simulink model "SMC_implementacion"  (R2024a)
settings: Solver=FixedStepAuto  StartTime=0.0  StopTime=inf  RelTol=1e-3  EnableMultiTasking=on
undefined symbols (not defined in the file): a, A_d, B_d, beta, C_d, L_d, theta_ref
libraries: arduinolib x2, eeLuenbergerObserver x1
settings Model: ExtModeTrigDuration=2  Creator=chris  LastModifiedBy=alfar
settings OptimizationCC: EnhancedBackFolding=on  PassReuseOutputArgsThreshold=0  MaxStackSize=64  OptimizeBlockOrder=speed  DifferentSizesBufferReuse=on  OptimizationCustomize=off
settings DebuggingCC: ParameterTunabilityLossMsg=error
settings HardwareCC: ProdBitPerInt=16  ProdBitPerPointer=16  ProdBitPerSizeT=16  ProdBitPerPtrDiffT=16  ProdLargestAtomicFloat=None  ProdWordSize=8  ProdHWDeviceType=Atmel->AVR  UseEmbeddedCoderFeatures=off  UseSimulinkCoderFeatures=off
settings SFSimCC: MATLABDynamicMemAlloc=off
settings RTWCC: Description=Embedded Coder  SystemTargetFile=ert.tlc  HardwareBoard=Arduino Mega 2560  TemplateMakefile=ert_default_tmf  RTWVerbose=off  Toolchain=Arduino AVR  BuildConfiguration=Faster Runs  GPUComputeCapability=3.5
settings CodeAppCC: ForceParamTrailComments=on  OperatorAnnotations=on  MangleLength=10
settings ERTTargetCC: ERTCustomFileBanners=off  SupportContinuousTime=on  SupportNonInlinedSFcns=on  RemoveResetFunc=off  SupportVariableSizeSignals=on  ModelStepFunctionPrototypeControlCompliant=off  ExtMode=on  ExtModeTransport=3  ExtModeStaticAlloc=on  ExtModeAutomaticAllocSize=off  ExtModeStaticAllocSize=2048  ExtModeMexFile=ext_xcp  ExtModeMexArgs=0 6 921600  ExtModeIntrfLevel=Level2 - Open  ERTSrcFileBannerTemplate=codertarget_code_template.cgt  ERTHdrFileBannerTemplate=codertarget_code_template.cgt  ERTDataSrcFileTemplate=codertarget_code_template.cgt  ERTDataHdrFileTemplate=codertarget_code_template.cgt

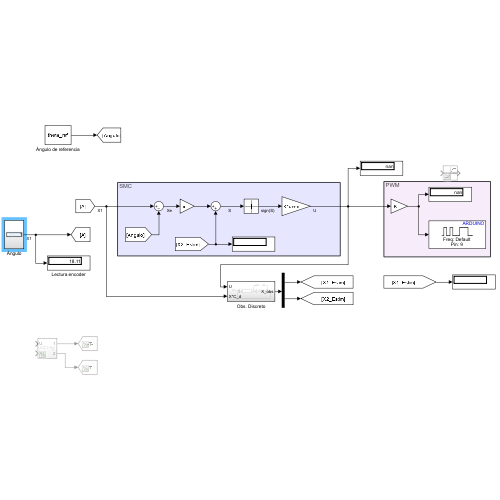
[thumbnail: Simulink's stored preview of the top-level diagram]
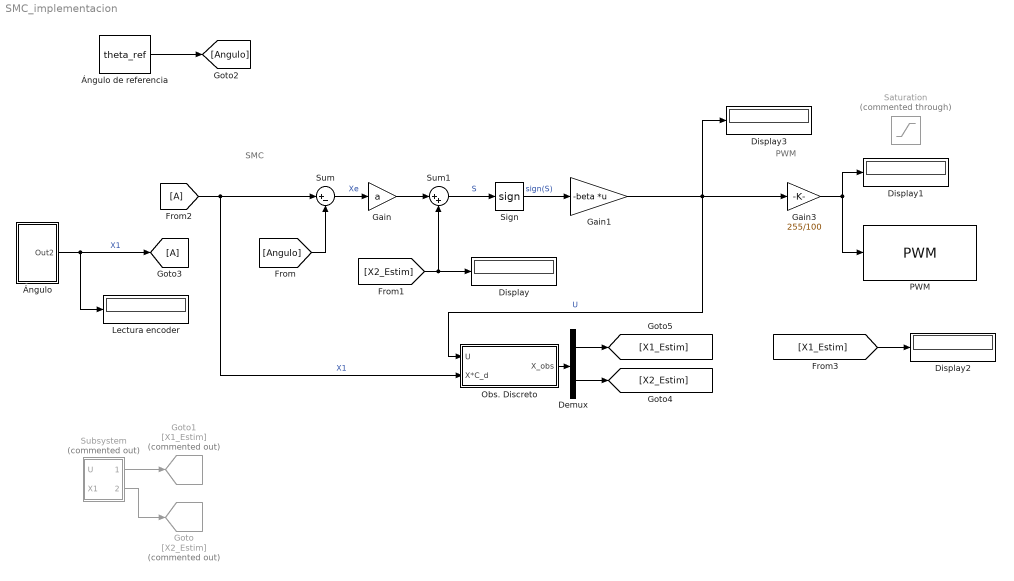
== system SMC_implementacion ==
  note: PWM
  note: SMC
  Demux : Demux  Outputs=2
  Display{,1..3} (4 alike) : Display
  From2 : From
  Gain : Gain  Gain=a
  Gain1 : Gain  Gain=-beta  Multiplication=Matrix(K*u) (u vector)
  Gain3 : Gain  Gain=255/100
  Goto : Goto  Commented=on  GotoTag=X2_Estim
  Goto1 : Goto  Commented=on  GotoTag=X1_Estim
  Goto3 : Goto
  Lectura encoder : Display
  Obs. Discreto : Subsystem
  PWM : arduinolib/PWM  pinNumber=9  frequencyType=Default  desiredFrequency=490.2  achievableFrequency=490.2
  Saturation : Saturate  Commented=through
  Sign : Signum  ZeroCross=off
  Subsystem : Subsystem  Commented=on
  Sum : Sum  Inputs=|+-
  Sum1 : Sum  Inputs=|++
  Ángulo : Subsystem
  Ángulo de referencia : Constant  Value=theta_ref
  wires:
  Sum/1 -> Gain/1  "Xe"
  Gain/1 -> Sum1/1
  [Angulo] -> Sum/2
  Sum1/1 -> Sign/1  "S"
  Sign/1 -> Gain1/1  "sign(S)"
  Ángulo de referencia/1 -> [Angulo]
  [X2_Estim] -> Display/1, Sum1/2
  Ángulo/1(Out2) -> Goto3/1, Lectura encoder/1  "X1"
  From2/1 -> Obs. Discreto/2(X*C_d), Sum/1  "X1"
  Subsystem/1(Out1) -> Goto1/1
  Subsystem/2(Out2) -> Goto/1
  Demux/1 -> [X1_Estim]
  Demux/2 -> [X2_Estim]
  Gain1/1 -> Obs. Discreto/1(U), Gain3/1, Display3/1  "U"
  Gain3/1 -> PWM/1, Display1/1
  Obs. Discreto/1(X_obs) -> Demux/1
  [X1_Estim] -> Display2/1

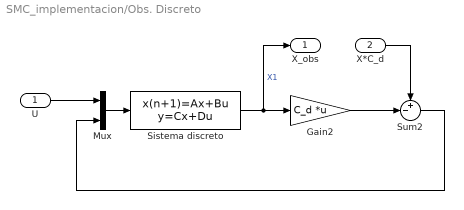
== system SMC_implementacion/Obs. Discreto ==
  U : Inport
  X*C_d : Inport  Port=2
  Gain2 : Gain  Gain=C_d  Multiplication=Matrix(K*u)
  Mux : Mux  Inputs=2
  Sistema discreto : DiscreteStateSpace  A=A_d  B=[B_d L_d]  C=eye(2)  D=zeros(2,2)  InitialCondition=[0; 0]  SampleTime=0.05
  Sum2 : Sum  Inputs=+-|
  X_obs : Outport
  wires:
  Gain2/1 -> Sum2/2
  Mux/1 -> Sistema discreto/1
  Sistema discreto/1 -> X_obs/1, Gain2/1  "X1"
  U/1 -> Mux/1
  X*C_d/1 -> Sum2/1
  Sum2/1 -> Mux/2

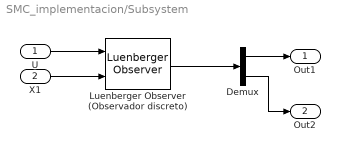
== system SMC_implementacion/Subsystem ==
  U : Inport
  X1 : Inport  Port=2
  Demux : Demux  Outputs=2
  Luenberger Observer (Observador discreto) : eeLuenbergerObserver/Luenberger Observer  StateSpaceType=Discrete-time  Ad=A_d  Bd=B_d  Cd=C_d  Dd=0  A=1  B=1  C=1  D=1  ObserverDesign=Observer gain  Ld=L_d  DesiredEigenvalues=0  x0=[0;0]  Tsd=0.1  Ts=0.01
      settings: LibrarySourceBlock=ee_sl_lib/Observers/Luenberger Observer
  Out1 : Outport
  Out2 : Outport  Port=2
  wires:
  X1/1 -> Luenberger Observer (Observador discreto)/2
  Demux/2 -> Out2/1
  U/1 -> Luenberger Observer (Observador discreto)/1
  Demux/1 -> Out1/1
  Luenberger Observer (Observador discreto)/1 -> Demux/1

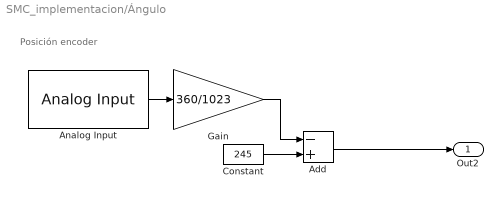
== system SMC_implementacion/Ángulo ==
  note: Posición encoder
  Add : Sum  Inputs=-+
  Analog Input : arduinolib/Analog Input  pinNumber=0  ReadResultsOnly=off  ConversionTriggerSource=Software  ExternalTriggerType=uint32( 0 )  OutputDataType=uint16  EnableConversionCompleteNotify=off  EnableOuputStatus=off  SampleTime=-1  blockPlatform=arduino
  Constant : Constant  Value=245
  Gain : Gain  Gain=360/1023
  Out2 : Outport
  wires:
  Analog Input/1 -> Gain/1
  Constant/1 -> Add/2
  Gain/1 -> Add/1
  Add/1 -> Out2/1
